simulink model "AI_Compare_2level"  (R2024b)
settings: Solver=ode1  StartTime=0.0  StopTime=4.5  FixedStep=Ts  RelTol=1e-3
PreLoadFcn:
  | Net_improve_init;L=Lac_MV;Tctrl=Ts;
PostLoadFcn:
  | Net_improve_init;L=Lac_MV;Tctrl=Ts;
InitFcn:
  | Net_improve_init;L=Lac_MV;Tctrl=Ts;
undefined symbols (not defined in the file or in its folder): C1, dend, DiscIntNeverNeededParam, f_cari, fs, Lac_MV, numd, Pref, R1, Rac_MV, Ts, Vac_peak_MV, Vdc
libraries: spsControlledVoltageSourceLib x28, powerlib_extras x25, spsGroundLib x14, spsControlledCurrentSourceLib x12, spsCurrentMeasurementLib x11, spsSeriesRLCBranchLib x7, spsThreePhaseVIMeasurementLib x6, spsIdealSwitchLib x5, spsPower3phInstantaneousLib x5, simulink x5, spsVoltageMeasurementLib x3, spsUniversalBridgeLib x1
(part 1 of 4)
Description:
  | The Model initialization function Callback automatically
  | 
  | sets the sample time  to 2e-6 sec.  and loads the initial
  | 
  | states vector xInitial. The initial state vector is saved in the
  | 
  | power_acdrive_init.mat file.
  | 
  | 
  | 
  | Check  the Initial state checkbox in the Simulation
  | 
  | parameters/Workspace I/O to start in steady state with a
  | 
  | speed of 120 rad/s and a torque of 0 N.m/s,
  | 
  | 
  | Copyright 2008-2015 The MathWorks, Inc.
settings Model: Creator=WeiLi  LastModifiedBy=KeXing
settings SolverCC: AlgebraicLoopSolver=TrustRegion
settings DataIOCC: SaveFinalState=on  SaveFormat=Array  SignalLoggingSaveFormat=ModelDataLogs  SaveOutput=off  SaveTime=off  SignalLoggingName=sigsOut
settings OptimizationCC: ExpressionDepthLimit=2147483647  InitFltsAndDblsToZero=on  LifeSpan=inf
settings DebuggingCC: ReadBeforeWriteMsg=DisableAll  WriteAfterWriteMsg=DisableAll  WriteAfterReadMsg=DisableAll  SaveWithParameterizedLinksMsg=none  UnderspecifiedInitializationDetection=Classic  MergeDetectMultiDrivingBlocksExec=none  CheckExecutionContextPreStartOutputMsg=on  MultiTaskDSMMsg=none  MultiTaskCondExecSysMsg=none  FcnCallInpInsideContextMsg=warning  UnconnectedInputMsg=warning  UnconnectedLineMsg=warning  StateNameClashWarn=warning  SFUnexpectedBacktrackingDiag=warning  SFNoUnconditionalDefaultTransitionDiag=warning  SFExecutionAtInitializationDiag=none  ArithmeticOperatorsInVariantConditions=warning
settings HardwareCC: ProdBitPerPointer=32  ProdBitPerSizeT=32  ProdBitPerPtrDiffT=32  ProdLargestAtomicFloat=None  ProdIntDivRoundTo=Undefined  ProdEndianess=Unspecified  ProdWordSize=32  ProdHWDeviceType=32-bit Generic  TargetUnknown=on
settings ModelReferenceCC: UpdateModelReferenceTargets=IfOutOfDate  EnableRefExpFcnMdlSchedulingChecks=on  PropagateSignalLabelsOutOfModel=off
settings SFSimCC: SFSimEcho=off  SimUseLocalCustomCode=off  CustomCodeUndefinedFunction=UseInterfaceOnly
settings RTWCC: RTWUseLocalCustomCode=off  GPUComputeCapability=3.5
settings CodeAppCC: StateflowObjectComments=on
settings GRTTargetCC: TargetFcnLib=ansi_tfl_tmw.mat  TargetLangStandard=C89/C90 (ANSI)  CombineOutputUpdateFcns=off  GRTInterface=on
settings ConfigComp: CovMetricSettings=dw  CovSaveCumulativeToWorkspaceVar=on  CovSaveSingleToWorkspaceVar=on  CovExternalEMLEnable=off
settings SimscapeCC: SimscapeNormalizeSystem=off

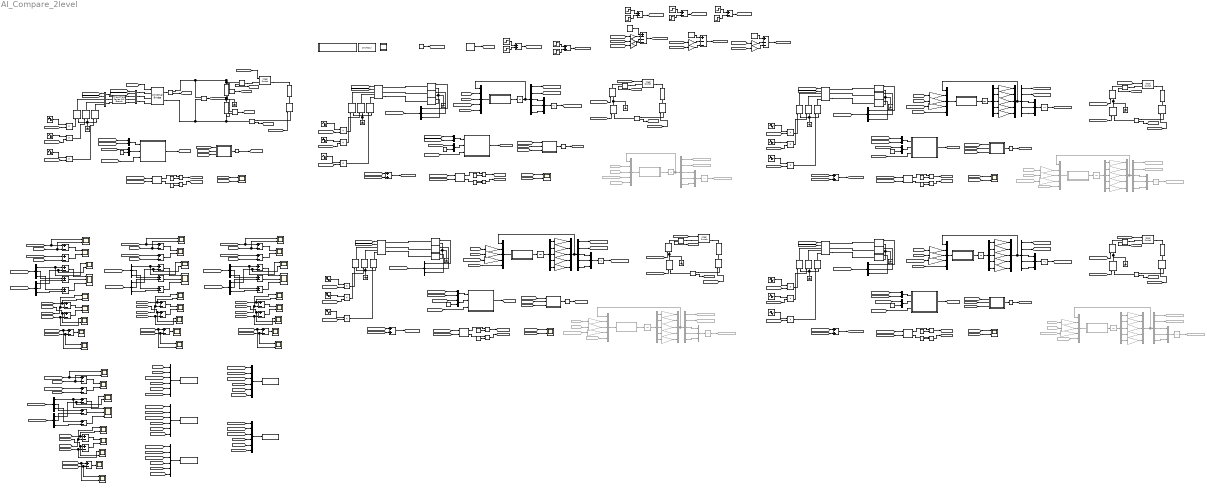
== system AI_Compare_2level ==
  note: Measurment
  note: Open-loop
  note: Close-loop
  note: pHNODE
  note: NODE
  note: Open-loop
  note: Close-loop
  note: pH-NODE vs DUB
  note: NODE vs DUB
  note: Open-loop
  note: LSTM
  note: Close-loop
  note: Close-loop
  note: PINODE
  note: Open-loop
  note: PINODE vs DUB
  note: LSTM vs DUB
  3fault_enable : Sum  Inputs=+-
  Bus_{1..6} (6 alike) : spsThreePhaseVIMeasurementLib/Three-Phase V-I Measurement  VoltageMeasurement=phase-to-ground  SetLabelV=off  LabelV=Vabc  Vpu=off  VpuLL=off  CurrentMeasurement=yes  SetLabelI=off  LabelI=Iabc  Ipu=off  Pbase=P_AC  Vbase=V_AC_prim  OutputType=Complex  PhasorSimulation=off  PSBequivalent=0
  Constant : Constant
  Constant1 : Constant
  Constant2 : Constant
  Controlled Current Source{1..12} (12 alike) : spsControlledCurrentSourceLib/Controlled Current Source  Initialize=on  Source_Type=AC  Amplitude=0  Phase=0  Frequency=0  Measurements=None
  Controlled Voltage Source{1..6,10,20..22,26..28} (13 alike) : spsControlledVoltageSourceLib/Controlled Voltage Source  Initialize=on  Source_Type=DC  Amplitude=3000  Phase=0  Frequency=0  Measurements=None
  Controlled Voltage Source{7..9,11..19,23..25} (15 alike) : spsControlledVoltageSourceLib/Controlled Voltage Source  Initialize=off  Source_Type=AC  Amplitude=0  Phase=0  Frequency=fs  Measurements=None
  Current Measurement{1..11} (11 alike) : spsCurrentMeasurementLib/Current Measurement  PhasorSimulation=off  OutputType=Complex  PSBequivalent=0
  Demux{,7,12,16,23..25} (7 alike) : Demux  Commented=on  Outputs=5
  Demux{1..3,5..6,8,13,17,19..22} (12 alike) : Demux  Outputs=3
  Demux{4,9..11,14..15,18} (7 alike) : Demux  Outputs=5
  Divide{1..10} (10 alike) : Product  Inputs=*/
  From115 : From  Commented=on  GotoTag=Idc_Ld5
  From117 : From  Commented=on  GotoTag=Idc_Ld6
  From119 : From  Commented=on  GotoTag=Vabc_Bus_MV3
  From{93,123,138,165} (4 alike) : From  Commented=on  GotoTag=pulses1
  From129 : From  Commented=on  GotoTag=Idc_Ld7
  From131 : From  Commented=on  GotoTag=Idc_Ld8
  From133 : From  Commented=on  GotoTag=Vabc_Bus_MV4
  From156 : From  Commented=on  GotoTag=Idc_Ld9
  From158 : From  Commented=on  GotoTag=Idc_Ld10
  From160 : From  Commented=on  GotoTag=Vabc_Bus_MV5
  From45 : From  Commented=on  GotoTag=Idc_Ld3
  From58 : From  Commented=on  GotoTag=Idc_Ld4
  From60 : From  Commented=on  GotoTag=Vabc_Bus_MV2
  Gain{,1..3} (4 alike) : Gain  Gain=0.9
  Gain10 : Gain  Gain=1811.85
  Gain11 : Gain  Gain=1795.81
  Gain12 : Gain  Gain=186.98
  Gain13 : Gain  Gain=193.63
  Gain14 : Gain  Gain=187.97
  Gain15 : Gain  Gain=1811.85
  Gain16 : Gain  Gain=1795.81
  Gain17 : Gain  Gain=186.98
  Gain18 : Gain  Gain=193.63
  Gain19 : Gain  Gain=187.97
  Gain{7,9,20,22,28,30} (6 alike) : Gain  Gain=1/116.32
  Gain21 : Gain  Gain=1/1405.94
  Gain23 : Gain  Commented=on  Gain=1811.85
  Gain24 : Gain  Commented=on  Gain=1795.81
  Gain25 : Gain  Commented=on  Gain=186.98
  Gain26 : Gain  Commented=on  Gain=193.63
  Gain27 : Gain  Commented=on  Gain=187.97
  Gain29 : Gain  Gain=1/1405.94
  Gain{31,33,39,41,47,49} (6 alike) : Gain  Commented=on  Gain=1/116.32
  Gain32 : Gain  Commented=on  Gain=1/1405.94
  Gain34 : Gain  Commented=on  Gain=1811.85
  Gain35 : Gain  Commented=on  Gain=1795.81
  Gain36 : Gain  Commented=on  Gain=186.98
  Gain37 : Gain  Commented=on  Gain=193.63
  Gain38 : Gain  Commented=on  Gain=187.97
  Gain4 : Gain  Gain=0.2
  Gain40 : Gain  Commented=on  Gain=1/1405.94
  Gain42 : Gain  Commented=on  Gain=1811.85
  Gain43 : Gain  Commented=on  Gain=1795.81
  Gain44 : Gain  Commented=on  Gain=186.98
  Gain45 : Gain  Commented=on  Gain=193.63
  Gain46 : Gain  Commented=on  Gain=187.97
  Gain48 : Gain  Commented=on  Gain=1/1405.94
  Gain5 : Gain  Gain=0.2
  Gain55 : Gain  Gain=1811.85
  Gain56 : Gain  Gain=1795.81
  Gain57 : Gain  Gain=186.98
  Gain58 : Gain  Gain=193.63
  Gain59 : Gain  Gain=187.97
  Gain6 : Gain  Gain=0.2
  Gain8 : Gain  Gain=1/1405.94
  Goto11 : Goto  Commented=on  GotoTag=Iabc_pred2
  Goto12 : Goto  Commented=on  GotoTag=vcp_pred3
  Goto13 : Goto  Commented=on  GotoTag=vcn_pred3
  Goto2 : Goto  Commented=on  GotoTag=Iabc_pred3
  Goto22 : Goto  Commented=on  GotoTag=vcp_pred2
  Goto23 : Goto  Commented=on  GotoTag=vcn_pred2
  Goto55 : Goto  Commented=on  GotoTag=Iabc_pred4
  Goto56 : Goto  Commented=on  GotoTag=vcp_pred4
  Goto61 : Goto  Commented=on  GotoTag=vcn_pred4
  Goto71 : Goto  Commented=on  GotoTag=Iabc_pred5
  Goto72 : Goto  Commented=on  GotoTag=vcp_pred5
  Goto76 : Goto  Commented=on  GotoTag=vcn_pred5
  Ground{1..14} (14 alike) : spsGroundLib/Ground  LConnTagsString=a
  Help : Subsystem  mask(OpDoc){docfile=../Help/help.html}
      mask init:
      | %patch([1,1,0,0,.8,1],[.8,0,0,1,1,.8],[.8 .8 .8]);
      | %patch([.15 .78 .78 .15 .15],[.8 .8 .83 .83 .8],[.9 .9 .9]);
      | %patch([.15 .78 .78 .15 .15],[.7 .7 .73 .73 .8],[.9 .9 .9]);
      | %patch([.15 .78 .78 .15 .15],[.6 .6 .63 .63 .6],[.9 .9 .9]);
      | %patch([.15 .78 .78 .15 .15],[.5 .5 .53 .53 .5],[.9 .9 .9]);
      | %patch([.15 .78 .78 .15 .15],[.4 .4 .43 .43 .4],[.9 .9 .9]);
      settings: OpenFcn=OpHelp_cb(gcb);
      mask Display: image(imread('opdoc.bmp'))
  IGBT Inverter2 : spsUniversalBridgeLib/Universal Bridge  Arms=3  SnubberResistance=IGBT_Rs  SnubberCapacitance=1e-6  Device=IGBT / Diodes  Ron=IGBT_Ron  Lon=0  ForwardVoltages=[0 0]  ForwardVoltage=.8  GTOparameters=[ 1e-6 , 1e-6 ]  IGBTparameters=[0 0]  Measurements=Device voltages  Measurements_2=None  converterType=Rectifier
      settings: AttributesFormatString=\n
  Ideal Switch{1..5} (5 alike) : spsIdealSwitchLib/Ideal Switch  Ron=0.001  Lon=0  IC=0  Rs=1e9  Cs=inf  Measurements=on
  Integrator : Integrator  Commented=on
  Integrator1 : Integrator
  Integrator2 : Integrator  Commented=on
  Integrator3 : Integrator  InitialCondition=1
  Integrator4 : Integrator  Commented=on
  Integrator7 : Integrator
  MATLAB Function : MATLAB Function  Commented=on  TreatAsAtomicUnit=on
  MATLAB Function1 : MATLAB Function  TreatAsAtomicUnit=on
  MATLAB Function2 : MATLAB Function  Commented=on  TreatAsAtomicUnit=on
  MATLAB Function3 : MATLAB Function  TreatAsAtomicUnit=on
  MATLAB Function4 : MATLAB Function  Commented=on  TreatAsAtomicUnit=on
  MATLAB Function5 : MATLAB Function  TreatAsAtomicUnit=on
  MATLAB Function6 : MATLAB Function  Commented=on  TreatAsAtomicUnit=on
  MATLAB Function7 : MATLAB Function  TreatAsAtomicUnit=on
  Memory{1..5} (5 alike) : Memory
  Minus{1..3,5} (4 alike) : Sum
  Model Initialization : Subsystem  mask(Model Functions){InitFcnX=Net_improve_init;L=Lac_MV;Tctrl=Ts;, prel=on, posl=on, inif=on, strf=off}
      mask prompts: InitFcnX "Initialisation"; prel "Preload Function"; posl "PostLoad Function"; inif "InitFcn"; strf "StartFcn"
      mask init:
      | currentBlock = gcb;
      | root = bdroot(currentBlock);
      | 
      | if ~strcmp(get_param(root,'BlockDiagramType'),'library')
      |     if prel==1
      |         set_param(root, 'PreLoadFcn', InitFcnX);
      |     else
      |         set_param(root, 'PreLoadFcn', '');
      |     end
      |     if inif==1
      |         set_param(root, 'InitFcn', InitFcnX);
      |     else
      |         set_param(root, 'InitFcn', '');
      |     end
      |     if strf==1
      |         set_param(root, 'StartFcn', InitFcnX);
      |     else
      |         set_param(root, 'StartFcn', '');
      |     end
      |     if posl==1
      |         set_param(root, 'PostLoadFcn', InitFcnX);
      |     else
      |         set_param(root, 'PostLoadFcn', '');
      |     end
      | end
      | 
      | pos = get_param(currentBlock, 'Position');
      | width = pos(3) - pos(1); height = pos(4) - pos(2);
      | txt = [ upper(root) '\n' '- InitFcn. . . . . '  get_param(root, 'InitFcn') ];
      settings: CopyFcn=set_param(gcb,'LinkStatus','none')
      mask Display: text(5, height*0.5, txt, 'horizontalAlignment', 'left', 'verticalAlignment', 'middle') ;
  Mux{,9,24,31} (4 alike) : Mux  Commented=on  Inputs=3
  Mux{1,10,18,25,34..36} (7 alike) : Mux  Commented=on  Inputs=5
  Mux{4..5,8,11,13..14,19..20,26..27} (10 alike) : Mux  Inputs=2
  Mux{2..3,12,32..33} (5 alike) : Mux  Inputs=6
  Mux{6,15,21,28} (4 alike) : Mux  Inputs=3
  Mux{7,16..17,22..23,29..30} (7 alike) : Mux  Inputs=5
  PWM_SPS1 : Subsystem
  PWM_SPS2 : Subsystem
  PWM_SPS3 : Subsystem
  PWM_SPS4 : Subsystem
  PWM_SPS5 : Subsystem
  P_AE{,1..3} (4 alike) : Sum  Inputs=+-
  Power (3ph, Instantaneous){1..5} (5 alike) : spsPower3phInstantaneousLib/Power (3ph, Instantaneous)
  Product{1..15} (15 alike) : Product
  Pstep : Sum
  Pstep1 : Sum
  Q_AE{,1..3} (4 alike) : Sum  Inputs=+-
  Qref_pu{1..5,7,10..11,13..14} (10 alike) : Constant  Value=Pref
  Qref_pu{6,8..9,12,15} (5 alike) : Constant  Value=0
  Rec_VQcontrol1 : Subsystem  mask(converter controller){cm=off, base=[Pref, Vac_peak_MV*sqrt(3/2), Vdc/2, fs], LRx=[Lac_MV, Rac_MV], LRx_inpu=off, Kd=[0.3  2]*10/6  %was [1 0.1]   ; [0.1  1]*1, Kp=[0.3 1]*1     %was [1 0.1]   ; [0.1  1]*1, Kvdc=[2 10]*1;   %was [0.5 1]*20 for Cdc=320uF, Vabc_lim=[-1 1], limitVdq=1.1, nadv=6, xtrIctrl1=[0.4 10 10 -10], Ts=Tctrl}
      mask prompts: cm "control mode (check VQ/uncheck PQ), only one terminal in VQ mode"; base "base value for power(VA), ac voltage(V), dc voltage to ground(V), and frequenvy(Hz) [Sb, Vb, Vdcb,freq]"; LRx "commutation inductance and resistance [Lx, Rx]"; LRx_inpu "[Lx, Rx] in pu if checked/ SI unchecked"; Kd "Kp Ki for d-axis PI control [kp ki]"; Kp "Kp Ki for q-axis PI control [kp ki]"; Kvdc "Kp Ki for Vdc PI control [kp ki]"; Vabc_lim "output Vabc limit [min max]"; limitVdq "limit for Vd,Vq (pu, default = 1.1)"; nadv "nb of time step to compesate for delay (default=1)"; xtrIctrl1 "[kp, kp, limitmax, limitmin] for current control (default=[0.4, 10, 10, -10])"
      mask help:
      | input 1, 6 dimentions, Vabc, Iabc, (SI)
      | input 2, 2 dimentions, Pref, Qref (PU)
      | input 3, 6 dimentions, Vcap at up arm a, lower arm a, up arm b, lower arm b, up arm c and lower arm c.
      | input 4, 1 dimention, pulse on
      | input 5, 1 dimention
      |
      | power or current directions: to go into grid is positive
      mask init:
      | if cm==0;
      |     x=['PQ\nmode'];
      | else
      |     x=['VQ\nmode'];
      | end
      | 
      | Sb=base(1);            %VA 3phase power base;
      | Vb=base(2);       %V, line-line rms voltage base
      | Ib=Sb/(sqrt(3)*Vb); %A, rms current base
      | Zb=Vb^2/Sb ;        %ohm, impedence base
      | Vdc=base(3);      %V Vdc+ to ground or ground to Vdc- 
      | frq=base(4);
      | 
      | if LRx_inpu
      |     Rxpu=LRx(2);
      |     Lxpu=LRx(1);
      | else
      |     Rxpu=LRx(2)/Zb;
      |     Lxpu=LRx(1)*2*pi*frq/Zb;
      | end;
      | 
      | ks=Vdc*sqrt(3/2)/Vb;     % ma=1/ks for 1pu dc ->1pu ac;
      | 
      | Kp=Kd;
      mask DialogControl ParameterTabVar0 Prompt: parameters
      mask DialogControl ParameterTabVar01 Prompt: advanced
      mask Display: disp (x);
  Rec_VQcontrol2 : Subsystem  mask(converter controller){cm=off, base=[Pref, Vac_peak_MV*sqrt(3/2), Vdc/2, fs], LRx=[Lac_MV, Rac_MV], LRx_inpu=off, Kd=[0.3  2]*10/6  %was [1 0.1]   ; [0.1  1]*1, Kp=[0.3 1]*1     %was [1 0.1]   ; [0.1  1]*1, Kvdc=[2 10]*1;   %was [0.5 1]*20 for Cdc=320uF, Vabc_lim=[-1 1], limitVdq=1.1, nadv=6, xtrIctrl1=[0.4 10 10 -10], Ts=Tctrl}
      mask prompts: cm "control mode (check VQ/uncheck PQ), only one terminal in VQ mode"; base "base value for power(VA), ac voltage(V), dc voltage to ground(V), and frequenvy(Hz) [Sb, Vb, Vdcb,freq]"; LRx "commutation inductance and resistance [Lx, Rx]"; LRx_inpu "[Lx, Rx] in pu if checked/ SI unchecked"; Kd "Kp Ki for d-axis PI control [kp ki]"; Kp "Kp Ki for q-axis PI control [kp ki]"; Kvdc "Kp Ki for Vdc PI control [kp ki]"; Vabc_lim "output Vabc limit [min max]"; limitVdq "limit for Vd,Vq (pu, default = 1.1)"; nadv "nb of time step to compesate for delay (default=1)"; xtrIctrl1 "[kp, kp, limitmax, limitmin] for current control (default=[0.4, 10, 10, -10])"
      mask help:
      | input 1, 6 dimentions, Vabc, Iabc, (SI)
      | input 2, 2 dimentions, Pref, Qref (PU)
      | input 3, 6 dimentions, Vcap at up arm a, lower arm a, up arm b, lower arm b, up arm c and lower arm c.
      | input 4, 1 dimention, pulse on
      | input 5, 1 dimention
      |
      | power or current directions: to go into grid is positive
      mask init: same as AI_Compare_2level/Rec_VQcontrol1
      mask DialogControl ParameterTabVar0 Prompt: parameters
      mask DialogControl ParameterTabVar01 Prompt: advanced
      mask Display: disp (x);
  Rec_VQcontrol3 : Subsystem  mask(converter controller){cm=off, base=[Pref, Vac_peak_MV*sqrt(3/2), Vdc/2, fs], LRx=[Lac_MV, Rac_MV], LRx_inpu=off, Kd=[0.3  2]*10/6  %was [1 0.1]   ; [0.1  1]*1, Kp=[0.3 1]*1     %was [1 0.1]   ; [0.1  1]*1, Kvdc=[2 10]*1;   %was [0.5 1]*20 for Cdc=320uF, Vabc_lim=[-1 1], limitVdq=1.1, nadv=6, xtrIctrl1=[0.4 10 10 -10], Ts=Tctrl}
      mask prompts: cm "control mode (check VQ/uncheck PQ), only one terminal in VQ mode"; base "base value for power(VA), ac voltage(V), dc voltage to ground(V), and frequenvy(Hz) [Sb, Vb, Vdcb,freq]"; LRx "commutation inductance and resistance [Lx, Rx]"; LRx_inpu "[Lx, Rx] in pu if checked/ SI unchecked"; Kd "Kp Ki for d-axis PI control [kp ki]"; Kp "Kp Ki for q-axis PI control [kp ki]"; Kvdc "Kp Ki for Vdc PI control [kp ki]"; Vabc_lim "output Vabc limit [min max]"; limitVdq "limit for Vd,Vq (pu, default = 1.1)"; nadv "nb of time step to compesate for delay (default=1)"; xtrIctrl1 "[kp, kp, limitmax, limitmin] for current control (default=[0.4, 10, 10, -10])"
      mask help:
      | input 1, 6 dimentions, Vabc, Iabc, (SI)
      | input 2, 2 dimentions, Pref, Qref (PU)
      | input 3, 6 dimentions, Vcap at up arm a, lower arm a, up arm b, lower arm b, up arm c and lower arm c.
      | input 4, 1 dimention, pulse on
      | input 5, 1 dimention
      |
      | power or current directions: to go into grid is positive
      mask init: same as AI_Compare_2level/Rec_VQcontrol1
      mask DialogControl ParameterTabVar0 Prompt: parameters
      mask DialogControl ParameterTabVar01 Prompt: advanced
      mask Display: disp (x);
  Rec_VQcontrol4 : Subsystem  mask(converter controller){cm=off, base=[Pref, Vac_peak_MV*sqrt(3/2), Vdc/2, fs], LRx=[Lac_MV, Rac_MV], LRx_inpu=off, Kd=[0.3  2]*10/6  %was [1 0.1]   ; [0.1  1]*1, Kp=[0.3 1]*1     %was [1 0.1]   ; [0.1  1]*1, Kvdc=[2 10]*1;   %was [0.5 1]*20 for Cdc=320uF, Vabc_lim=[-1 1], limitVdq=1.1, nadv=6, xtrIctrl1=[0.4 10 10 -10], Ts=Tctrl}
      mask prompts: cm "control mode (check VQ/uncheck PQ), only one terminal in VQ mode"; base "base value for power(VA), ac voltage(V), dc voltage to ground(V), and frequenvy(Hz) [Sb, Vb, Vdcb,freq]"; LRx "commutation inductance and resistance [Lx, Rx]"; LRx_inpu "[Lx, Rx] in pu if checked/ SI unchecked"; Kd "Kp Ki for d-axis PI control [kp ki]"; Kp "Kp Ki for q-axis PI control [kp ki]"; Kvdc "Kp Ki for Vdc PI control [kp ki]"; Vabc_lim "output Vabc limit [min max]"; limitVdq "limit for Vd,Vq (pu, default = 1.1)"; nadv "nb of time step to compesate for delay (default=1)"; xtrIctrl1 "[kp, kp, limitmax, limitmin] for current control (default=[0.4, 10, 10, -10])"
      mask help:
      | input 1, 6 dimentions, Vabc, Iabc, (SI)
      | input 2, 2 dimentions, Pref, Qref (PU)
      | input 3, 6 dimentions, Vcap at up arm a, lower arm a, up arm b, lower arm b, up arm c and lower arm c.
      | input 4, 1 dimention, pulse on
      | input 5, 1 dimention
      |
      | power or current directions: to go into grid is positive
      mask init: same as AI_Compare_2level/Rec_VQcontrol1
      mask DialogControl ParameterTabVar0 Prompt: parameters
      mask DialogControl ParameterTabVar01 Prompt: advanced
      mask Display: disp (x);
  Rec_VQcontrol5 : Subsystem  mask(converter controller){cm=off, base=[Pref, Vac_peak_MV*sqrt(3/2), Vdc/2, fs], LRx=[Lac_MV, Rac_MV], LRx_inpu=off, Kd=[0.3  2]*10/6  %was [1 0.1]   ; [0.1  1]*1, Kp=[0.3 1]*1     %was [1 0.1]   ; [0.1  1]*1, Kvdc=[2 10]*1;   %was [0.5 1]*20 for Cdc=320uF, Vabc_lim=[-1 1], limitVdq=1.1, nadv=6, xtrIctrl1=[0.4 10 10 -10], Ts=Tctrl}
      mask prompts: cm "control mode (check VQ/uncheck PQ), only one terminal in VQ mode"; base "base value for power(VA), ac voltage(V), dc voltage to ground(V), and frequenvy(Hz) [Sb, Vb, Vdcb,freq]"; LRx "commutation inductance and resistance [Lx, Rx]"; LRx_inpu "[Lx, Rx] in pu if checked/ SI unchecked"; Kd "Kp Ki for d-axis PI control [kp ki]"; Kp "Kp Ki for q-axis PI control [kp ki]"; Kvdc "Kp Ki for Vdc PI control [kp ki]"; Vabc_lim "output Vabc limit [min max]"; limitVdq "limit for Vd,Vq (pu, default = 1.1)"; nadv "nb of time step to compesate for delay (default=1)"; xtrIctrl1 "[kp, kp, limitmax, limitmin] for current control (default=[0.4, 10, 10, -10])"
      mask help:
      | input 1, 6 dimentions, Vabc, Iabc, (SI)
      | input 2, 2 dimentions, Pref, Qref (PU)
      | input 3, 6 dimentions, Vcap at up arm a, lower arm a, up arm b, lower arm b, up arm c and lower arm c.
      | input 4, 1 dimention, pulse on
      | input 5, 1 dimention
      |
      | power or current directions: to go into grid is positive
      mask init: same as AI_Compare_2level/Rec_VQcontrol1
      mask DialogControl ParameterTabVar0 Prompt: parameters
      mask DialogControl ParameterTabVar01 Prompt: advanced
      mask Display: disp (x);
  Scope{1..2,4..9,11..13,15..19,21..23,25..27,29..32,34..36,38..41} (33 alike) : Scope  NumInputPorts=2
  Scope{10,14,24,33} (4 alike) : Scope
  Scope{3,20,28,37} (4 alike) : Scope  NumInputPorts=3
  Series RLC Branch{1..2,4,6..7} (5 alike) : spsSeriesRLCBranchLib/Series RLC Branch  LConnTagsString=__new0  RConnTagsString=__new0  BranchType=R  Resistance=3e3^2/(Pref)/10*2  Inductance=1e-3  SetiL0=off  InitialCurrent=0  Capacitance=C1  Setx0=off  InitialVoltage=0  Measurements=None
  Series RLC Branch3 : spsSeriesRLCBranchLib/Series RLC Branch  LConnTagsString=__new0  RConnTagsString=__new0  BranchType=C  Resistance=R1  Inductance=1e-3  SetiL0=off  InitialCurrent=0  Capacitance=C1  Setx0=off  InitialVoltage=0  Measurements=None
  Series RLC Branch5 : spsSeriesRLCBranchLib/Series RLC Branch  LConnTagsString=__new0  RConnTagsString=__new0  BranchType=C  Resistance=R1  Inductance=1e-3  SetiL0=off  InitialCurrent=0  Capacitance=C1  Setx0=off  InitialVoltage=0  Measurements=None
  Sine Wave{1,3,6,10,13} (5 alike) : Sin  Amplitude=3e3/2*sqrt(2/3)  Frequency=2*pi*fs  SampleTime=0
  Sine Wave{2,4,7,11,14} (5 alike) : Sin  Amplitude=3e3/2*sqrt(2/3)  Frequency=2*pi*fs  Phase=-2*pi/3  SampleTime=0
  Sine Wave{5,8..9,12,15} (5 alike) : Sin  Amplitude=3e3/2*sqrt(2/3)  Frequency=2*pi*fs  Phase=+2*pi/3  SampleTime=0
  Step1 : Step  Time=2.75  Before=-0.8  After=-0.6  SampleTime=0
  Step10 : Step  Time=3.85  SampleTime=0
  Step2 : Step  Time=3.25  Before=3000  After=2400  SampleTime=0
  Step3 : Step  Time=3.0  Before=0.0  After=-0.2  SampleTime=0
  Step4 : Step  Time=1.75  Before=1.9  SampleTime=0
  Step5 : Step  Time=3.5  After=600  SampleTime=0
  Step6 : Step  Time=1.65  SampleTime=0
  Step7 : Step  Time=2.5  SampleTime=0
  Step8 : Step  Time=2.65  SampleTime=0
  Step9 : Step  Time=3.70  SampleTime=0
  Three-Phase RL1 : spsThreePhaseSeriesRLCBranchLib/Three-Phase Series RLC Branch  LConnTagsString=A|B|C  RConnTagsString=A|B|C  BranchType=RL  Resistance=Rac_MV  Inductance=Lac_MV  Capacitance=1e-6  Measurements=None
  To Workspace : ToWorkspace  VariableName=z_pq_phnode  SampleTime=-1
      settings: Save2DSignal=2-D array (concatenate along first dimension)
  To Workspace1 : ToWorkspace  VariableName=z_pq_dub  SampleTime=-1
      settings: Save2DSignal=2-D array (concatenate along first dimension)
  To Workspace2 : ToWorkspace  VariableName=z_pq_node  SampleTime=-1
      settings: Save2DSignal=2-D array (concatenate along first dimension)
  To Workspace3 : ToWorkspace  VariableName=z_pq_lstm  SampleTime=-1
      settings: Save2DSignal=2-D array (concatenate along first dimension)
  To Workspace4 : ToWorkspace  VariableName=z_pq_pinode  SampleTime=-1
      settings: Save2DSignal=2-D array (concatenate along first dimension)
  Unary Minus{1,3,5,7} (4 alike) : UnaryMinus  Commented=on
  Unary Minus{2,4,6,8} (4 alike) : UnaryMinus
  Unit Delay : UnitDelay  SampleTime=-1  HasFrameUpgradeWarning=on
  Unit Delay1 : UnitDelay  Commented=on  SampleTime=-1  HasFrameUpgradeWarning=on
  Voltage Measurement1 : spsVoltageMeasurementLib/Voltage Measurement  PhasorSimulation=off  OutputType=Complex  PSBequivalent=0
  Voltage Measurement2 : spsVoltageMeasurementLib/Voltage Measurement  PhasorSimulation=off  OutputType=Complex  PSBequivalent=0
  Voltage Measurement3 : spsVoltageMeasurementLib/Voltage Measurement  PhasorSimulation=off  OutputType=Complex  PSBequivalent=0
  afault_enable1 : Sum  Inputs=+-
  afault_enable2 : Sum  Inputs=+-
  carrier gen1 : libMMCcpuv2/carrier gen  fc=f_cari*2  range=[ 1 -1]  Ms=3  Ns=1
  ia_AE{,1..3} (4 alike) : Sum  Inputs=+-
  ib_AE{,1..3} (4 alike) : Sum  Inputs=+-
  ic_AE{,1..3} (4 alike) : Sum  Inputs=+-
  ka : Sum  Inputs=+---
  kb : Sum  Inputs=+--
  kb1 : Sum  Inputs=+--
  powergui : spspowerguiLib/powergui  Priority=2  SimulationMode=Discrete  SampleTime=Ts  frequency=60  Iterations=50  frequencyindice=0  Pbase=100e6  ErrMax=1e-4  UnitsV=kV  UnitsW=MW  buscounter=0  FunctionMessages=off  echomessages=off  EnableUseOfTLC=off  CurrentSourceSwitches=off  DisableSnubberDevices=off  DisableRonSwitches=off  DisableVfSwitches=off  DisplayEquations=off  AutomaticDiscreteSolvers=off  SolverType=Backward Euler  Interpol=off  ExternalGateDelay=off  methode=off  Ts=0  x0status=blocks  SPID=off  SwTol=0  HookPort=off  NonlinearTolerance=1e-4  nMaxIteration=100  ContinueOnMaxIteration=off  RestoreLinks=warning  ResistiveCurrentMeasurement=off  Frange=[0:2:500]  Ylog=off  Xlog=on  ShowGrid=off  save=off  variable=ZData  structure=VI  ZoomFFT=off  StartTime=9  cycles=10  DisplayStyle=2  fundamental=300/pi  FreqAxis=off  MaxFrequency=1000  frequencyindicesteady=1  RmsSteady=1  display=off
  pulse_enable : Constant
  vcn_AE{,1..3} (4 alike) : Sum  Inputs=+-
  vcp_AE{,1..7} (8 alike) : Sum  Inputs=+-
  wires:
  carrier gen1/1 -> [pwmcarrier]
  [pulse_enable] -> PWM_SPS3/1(enable)
  Mux4/1 -> Rec_VQcontrol2/1(meas)
  Mux5/1 -> Rec_VQcontrol2/2(PQref)
  Qref_pu6/1 -> Mux5/2
  [power_step] -> Mux5/1
  pulse_enable/1 -> [pulse_enable]
  PWM_SPS3/1(Pulse) -> Memory2/1
  Rec_VQcontrol2/1(V_cell_ref) -> [Vref_PQctrl2]
  Memory2/1 -> [pulses2]
  [Iabc_Bus_MV1] -> Demux1/1
  vcp_AE/1 -> Scope2/1
  vcn_AE/1 -> Scope2/2
  ib_AE/1 -> Scope3/2
  ic_AE/1 -> Scope3/3
  Step1/1 -> Pstep/1
  Bus_2/1 -> [Vabc_Bus_MV2]
  Bus_2/2 -> [Iabc_Bus_MV2]
  [pulse_enable] -> Ideal Switch1/1
  Current Measurement2/1 -> [Idc_Ld3]
  Current Measurement4/1 -> [Idc_Ld4]
  [vcp_pred2] -> Controlled Voltage Source1/1
  [vcn_pred2] -> Controlled Voltage Source5/1
  Minus5/1 -> [Vdc_pred2]
  [vcp_pred2] -> Minus5/1
  [vcn_pred2] -> Minus5/2
  Demux1/2 -> ib_AE/2
  Demux1/3 -> ic_AE/2
  Demux3/1 -> Scope13/1, ia_AE/1
  Demux3/2 -> ib_AE/1
  Demux3/3 -> ic_AE/1
  [Iabc_pred2] -> Demux3/1
  [Vcp1] -> Scope4/2, vcp_AE/2
  [Vcn1] -> vcn_AE/2
  [vcp_pred2] -> Scope4/1, vcp_AE/1
  [vcn_pred2] -> vcn_AE/1
  "Power (3ph, Instantaneous)1"/1 -> Divide2/1
  Qref_pu4/1 -> Divide3/2
  Qref_pu3/1 -> Divide2/2
  "Power (3ph, Instantaneous)1"/2 -> Divide3/1
  Divide2/1 -> [P2]
  Divide3/1 -> [Q2]
  [P2] -> Scope8/1
  [Q2] -> Scope8/2
  [Vabc_Bus_MV2] -> "Power (3ph, Instantaneous)1"/1
  [Iabc_Bus_MV2] -> "Power (3ph, Instantaneous)1"/2
  Integrator/1 -> Mux1/1, Demux/1
  [Iabc_pred2] -> Demux2/1
  Demux2/1 -> Controlled Current Source2/1
  Demux2/2 -> Controlled Current Source1/1
  Demux2/3 -> Controlled Current Source3/1
  [P1] -> Scope11/2, P_AE/1
  [P2] -> P_AE/2, Scope11/1
  [Q1] -> Scope17/2, Q_AE/1
  [Q2] -> Scope17/1, Q_AE/2
  P_AE/1 -> Scope1/1
  Q_AE/1 -> Scope1/2
  ia_AE/1 -> Scope3/1
  Demux1/1 -> Scope13/2, ia_AE/2
  [vcp_pred2] -> Mux2/1
  [vcn_pred2] -> Mux2/2
  [Iabc_pred2] -> Mux2/3
  [P2] -> Mux2/4
  [Q2] -> Mux2/5
  Mux2/1 -> To Workspace/1
  [Vcp1] -> Mux3/1
  [Vcn1] -> Mux3/2
  [Iabc_Bus_MV1] -> Mux3/3
  [P1] -> Mux3/4
  [Q1] -> Mux3/5
  Mux3/1 -> To Workspace1/1
  [Idc_Ld3] -> Mux7/2
  Integrator1/1 -> Mux7/1, Demux4/1
  [Idc_Ld4] -> Mux7/3
  Demux4/2 -> [vcn_pred2]  "vcn"
  Unary Minus2/1 -> [Iabc_pred2]
  MATLAB Function1/1(dz) -> Integrator1/1
  [Vabc_Bus_MV2] -> Mux7/4
  Mux7/1 -> MATLAB Function1/1(u)
  Demux4/5 -> Mux6/3  "ic"
  Mux6/1 -> Unary Minus2/1
  Demux4/1 -> [vcp_pred2]  "vcp"
  Demux4/4 -> Mux6/2  "ib"
  Demux4/3 -> Mux6/1  "ia"
  From45/1 -> Mux1/2
  From58/1 -> Mux1/3
  From60/1 -> Mux1/4
  From93/1 -> Mux1/5
  MATLAB Function/1(dz) -> Integrator/1
  Demux/1 -> Goto22/1  "vcp"
  Demux/2 -> Goto23/1  "vcn"
  Demux/3 -> Mux/1  "ia"
  Demux/4 -> Mux/2  "ib"
  Demux/5 -> Mux/3  "ic"
  Mux/1 -> Unary Minus1/1
  Unary Minus1/1 -> Goto11/1
  Mux1/1 -> MATLAB Function/1(u)
  [dc_step] -> Controlled Voltage Source2/1
  Sine Wave5/1 -> Product5/1
  Sine Wave3/1 -> Product3/1
  [ac_step_c] -> Product5/2
  Sine Wave4/1 -> Product4/1
  [ac_step_b] -> Product4/2
  [ac_step_a] -> Product3/2
  Product3/1 -> Controlled Voltage Source7/1
  Product4/1 -> Controlled Voltage Source8/1
  Product5/1 -> Controlled Voltage Source9/1
  [Iabc_Bus_MV2] -> Mux4/2
  [Vref_PQctrl2] -> PWM_SPS3/2(Vref)
  [pwmcarrier] -> PWM_SPS3/3(pwmcarrier)
  [Vabc_Bus_MV2] -> Mux4/1
  [Vdc_pred2] -> Rec_VQcontrol2/3(Vdc)
  [Vdc_pred2] -> Scope15/2, vcp_AE6/1
  [Vdc_meas1] -> Scope15/1, vcp_AE6/2
  vcp_AE6/1 -> Scope14/1
  [Vdc_pred2] -> Mux2/6
  [Vdc_meas1] -> Mux3/6
  [pulses2] -> Mux7/5
  [Vabc_Bus_MV1] -> "Power (3ph, Instantaneous)2"/1
  Qref_pu7/1 -> Divide5/2
  [Iabc_Bus_MV1] -> "Power (3ph, Instantaneous)2"/2
  Mux8/1 -> Rec_VQcontrol3/2(PQref)
  Divide5/1 -> [Q1]
  Rec_VQcontrol3/1(V_cell_ref) -> [Vref_PQctrl1]
  [power_step] -> Mux8/1
  Voltage Measurement1/1 -> [Vcp1]
  Sine Wave7/1 -> Product7/1
  Qref_pu9/1 -> Mux8/2
  [dc_step] -> Controlled Voltage Source10/1
  Voltage Measurement3/1 -> [Vdc_meas1]
  [Iabc_Bus_MV1] -> Mux11/2
  Sine Wave8/1 -> Product8/1
  Memory3/1 -> [pulses1]
  [P1] -> Scope12/1
  Bus_5/1 -> [Vabc_con_MV1]
  Current Measurement8/1 -> [Idc_Ld2]
  Voltage Measurement2/1 -> [Vcn1]
  Sine Wave6/1 -> Product6/1
  Product6/1 -> Controlled Voltage Source11/1
  [pulses1] -> IGBT Inverter2/1
  Bus_3/2 -> [Iabc_Bus_MV1]
  [Vabc_Bus_MV1] -> Mux11/1
  [ac_step_c] -> Product8/2
  [pulse_enable] -> PWM_SPS2/1(enable)
  [Vdc_meas1] -> Rec_VQcontrol3/3(Vdc)
  Current Measurement6/1 -> [Idc_meas1]
  Mux11/1 -> Rec_VQcontrol3/1(meas)
  [ac_step_b] -> Product7/2
  "Power (3ph, Instantaneous)2"/2 -> Divide5/1
  [pwmcarrier] -> PWM_SPS2/3(pwmcarrier)
  [pulse_enable] -> Ideal Switch3/1
  Current Measurement7/1 -> [Idc_Ld1]
  Product8/1 -> Controlled Voltage Source13/1
  "Power (3ph, Instantaneous)2"/1 -> Divide4/1
  [Q1] -> Scope12/2
  [Vref_PQctrl1] -> PWM_SPS2/2(Vref)
  Divide4/1 -> [P1]
  Qref_pu5/1 -> Divide4/2
  Bus_3/1 -> [Vabc_Bus_MV1]
  Bus_5/2 -> [iabc_con_MV1]
  [ac_step_a] -> Product6/2
  Product7/1 -> Controlled Voltage Source12/1
  PWM_SPS2/1(Pulse) -> Memory3/1
  [P1] -> Scope7/2, P_AE1/1
  P_AE1/1 -> Scope5/1
  vcn_AE1/1 -> Scope19/2
  Demux6/1 -> Scope9/1, ia_AE1/1
  Demux5/1 -> Scope9/2, ia_AE1/2
  Demux5/3 -> ic_AE1/2
  Demux5/2 -> ib_AE1/2
  [Q1] -> Scope18/2, Q_AE1/1
  vcp_AE1/1 -> Scope19/1
  [Iabc_pred3] -> Demux6/1
  [Iabc_Bus_MV1] -> Demux5/1
  ic_AE1/1 -> Scope20/3
  Demux6/2 -> ib_AE1/1
  ia_AE1/1 -> Scope20/1
  vcp_AE2/1 -> Scope10/1
  [Q3] -> Scope18/1, Q_AE1/2
  Q_AE1/1 -> Scope5/2
  [P3] -> P_AE1/2, Scope7/1
  [Vcp1] -> Scope21/2, vcp_AE1/2
  [vcp_pred3] -> Scope21/1, vcp_AE1/1
  [vcn_pred3] -> vcn_AE1/1
  Demux6/3 -> ic_AE1/1
  [Vdc_meas1] -> Scope16/1, vcp_AE2/2
  [Vcn1] -> vcn_AE1/2
  [Vdc_pred3] -> Scope16/2, vcp_AE2/1
  ib_AE1/1 -> Scope20/2
  Step2/1 -> Pstep1/1
  Step4/1 -> 3fault_enable/1
  Step6/1 -> 3fault_enable/2
  Step7/1 -> afault_enable1/1
  Step8/1 -> afault_enable1/2
  3fault_enable/1 -> [enable_3fault]
  afault_enable1/1 -> [enable_afault]
  ka/1 -> [ac_step_a]
  [enable_3fault] -> Gain/1
  Gain/1 -> ka/2
  [enable_afault] -> Gain1/1
  Gain1/1 -> ka/3
  Constant/1 -> ka/1
  kb/1 -> [ac_step_b]
  Constant1/1 -> kb/1
  [enable_3fault] -> Gain2/1
  Gain2/1 -> kb/2
  Step3/1 -> Pstep/2
  Pstep/1 -> [power_step]
  Pstep1/1 -> [dc_step]
  Step5/1 -> Pstep1/2
  Step9/1 -> afault_enable2/1
  Step10/1 -> afault_enable2/2
  afault_enable2/1 -> [enable_edisturb]
  Gain4/1 -> ka/4
  [enable_edisturb] -> Gain4/1
  [enable_edisturb] -> Gain5/1
  Gain5/1 -> kb/3
  [enable_3fault] -> Gain3/1
  Gain3/1 -> kb1/2
  Gain6/1 -> kb1/3
  [enable_edisturb] -> Gain6/1
  kb1/1 -> [ac_step_c]
  Constant2/1 -> kb1/1
  PWM_SPS1/1(Pulse) -> Memory1/1
  Mux16/1 -> MATLAB Function3/1(u)
  [Iabc_Bus_MV3] -> Mux13/2
  [Vabc_Bus_MV3] -> Gain8/1
  Memory1/1 -> [pulses3]
  Product9/1 -> Controlled Voltage Source16/1
  [Iabc_pred3] -> Demux8/1
  [Vref_PQctrl3] -> PWM_SPS1/2(Vref)
  [vcp_pred3] -> Minus1/1
  Bus_1/1 -> [Vabc_Bus_MV3]
  Sine Wave2/1 -> Product2/1
  [pulse_enable] -> Ideal Switch2/1
  Demux9/5 -> Mux15/3  "ic"
  Rec_VQcontrol1/1(V_cell_ref) -> [Vref_PQctrl3]
  Sine Wave9/1 -> Product9/1
  Current Measurement1/1 -> [Idc_Ld5]
  Unary Minus4/1 -> [Iabc_pred3]
  Qref_pu8/1 -> Mux14/2
  Divide6/1 -> [Q3]
  [vcp_pred3] -> Controlled Voltage Source3/1
  [Vdc_pred3] -> Rec_VQcontrol1/3(Vdc)
  [Vabc_Bus_MV3] -> "Power (3ph, Instantaneous)3"/1
  Current Measurement3/1 -> [Idc_Ld6]
  [ac_step_a] -> Product1/2
  [pulse_enable] -> PWM_SPS1/1(enable)
  Demux8/2 -> Controlled Current Source4/1
  [power_step] -> Mux14/1
  [pwmcarrier] -> PWM_SPS1/3(pwmcarrier)
  "Power (3ph, Instantaneous)3"/2 -> Divide6/1
  Demux9/4 -> Mux15/2  "ib"
  [pulses3] -> Mux16/5
  Mux10/1 -> MATLAB Function2/1(u)
  Qref_pu1/1 -> Divide1/2
  Mux14/1 -> Rec_VQcontrol1/2(PQref)
  [ac_step_c] -> Product9/2
  Demux8/1 -> Controlled Current Source5/1
  [Vabc_Bus_MV3] -> Mux13/1
  Minus1/1 -> [Vdc_pred3]
  Qref_pu2/1 -> Divide6/2
  From115/1 -> Gain31/1
  Sine Wave1/1 -> Product1/1
  "Power (3ph, Instantaneous)3"/1 -> Divide1/1
  [Idc_Ld5] -> Gain7/1
  From123/1 -> Mux10/5
  Divide1/1 -> [P3]
  [Q3] -> Scope6/2
  Bus_1/2 -> [Iabc_Bus_MV3]
  [Idc_Ld6] -> Gain9/1
  Demux9/1 -> [vcp_pred3]  "vcp"
  [dc_step] -> Controlled Voltage Source4/1
  Mux13/1 -> Rec_VQcontrol1/1(meas)
  [ac_step_b] -> Product2/2
  [Iabc_Bus_MV3] -> "Power (3ph, Instantaneous)3"/2
  [vcn_pred3] -> Controlled Voltage Source6/1
  From117/1 -> Gain33/1
  Demux9/3 -> Mux15/1  "ia"
  Mux15/1 -> Unary Minus4/1
  MATLAB Function3/1(dz) -> Integrator3/1
  [vcn_pred3] -> Minus1/2
  [P3] -> Scope6/1
  Demux8/3 -> Controlled Current Source6/1
  Product1/1 -> Controlled Voltage Source14/1
  From119/1 -> Gain32/1
  Demux9/2 -> [vcn_pred3]  "vcn"
  Product2/1 -> Controlled Voltage Source15/1
  [Q3] -> Mux12/5
  [Iabc_pred3] -> Mux12/3
  [vcp_pred3] -> Mux12/1
  [Vdc_pred3] -> Mux12/6
  [P3] -> Mux12/4
  [vcn_pred3] -> Mux12/2
  Mux12/1 -> To Workspace2/1
  Gain7/1 -> Mux16/2
  Gain9/1 -> Mux16/3
  Gain8/1 -> Mux16/4
  Integrator3/1 -> Demux10/1
  Demux10/1 -> Gain10/1  "vcp"
  Demux10/2 -> Gain11/1  "vcn"
  Demux10/3 -> Gain12/1  "ia"
  Demux10/4 -> Gain13/1  "ib"
  Demux10/5 -> Gain14/1  "ic"
  Gain10/1 -> Mux17/1
  Gain11/1 -> Mux17/2
  Gain12/1 -> Mux17/3
  Gain13/1 -> Mux17/4
  Gain14/1 -> Mux17/5
  Mux17/1 -> Mux16/1, Demux9/1
  Gain22/1 -> Mux22/3
  [Idc_Ld8] -> Gain22/1
  Demux13/1 -> Controlled Current Source8/1
  [Vabc_Bus_MV4] -> Mux19/1
  [ac_step_c] -> Product12/2
  From129/1 -> Gain39/1
  Qref_pu11/1 -> Divide8/2
  Minus2/1 -> [Vdc_pred4]
  Mux23/1 -> Mux22/1, Demux14/1
  Gain20/1 -> Mux22/2
  "Power (3ph, Instantaneous)4"/2 -> Divide8/1
  Mux18/1 -> MATLAB Function4/1(u)
  Mux20/1 -> Rec_VQcontrol4/2(PQref)
  Bus_4/2 -> [Iabc_Bus_MV4]
  [Q4] -> Scope22/2
  From133/1 -> Gain40/1
  [P4] -> Scope22/1
  Product10/1 -> Controlled Voltage Source17/1
  Demux13/3 -> Controlled Current Source9/1
  [vcn_pred4] -> Minus2/2
  From131/1 -> Gain41/1
  [ac_step_b] -> Product11/2
  Mux19/1 -> Rec_VQcontrol4/1(meas)
  [dc_step] -> Controlled Voltage Source21/1
  [Idc_Ld7] -> Gain20/1
  "Power (3ph, Instantaneous)4"/1 -> Divide7/1
  Sine Wave10/1 -> Product10/1
  From138/1 -> Mux18/5
  PWM_SPS4/1(Pulse) -> Memory4/1
  Demux13/2 -> Controlled Current Source7/1
  [pulse_enable] -> PWM_SPS4/1(enable)
  Current Measurement9/1 -> [Idc_Ld8]
  [pwmcarrier] -> PWM_SPS4/3(pwmcarrier)
  [power_step] -> Mux20/1
  Qref_pu12/1 -> Mux20/2
  [vcp_pred4] -> Controlled Voltage Source20/1
  Product11/1 -> Controlled Voltage Source18/1
  Rec_VQcontrol4/1(V_cell_ref) -> [Vref_PQctrl4]
  Current Measurement5/1 -> [Idc_Ld7]
  [Vref_PQctrl4] -> PWM_SPS4/2(Vref)
  [Vabc_Bus_MV4] -> Gain21/1
  Bus_4/1 -> [Vabc_Bus_MV4]
  Gain21/1 -> Mux22/4
  Product12/1 -> Controlled Voltage Source19/1
  Qref_pu10/1 -> Divide7/2
  Sine Wave11/1 -> Product11/1
  [vcp_pred4] -> Minus2/1
  [vcn_pred4] -> Controlled Voltage Source22/1
  Memory4/1 -> [pulses4]
  [Iabc_pred4] -> Demux13/1
  [pulses4] -> Mux22/5
  [Iabc_Bus_MV4] -> Mux19/2
  [Vdc_pred4] -> Rec_VQcontrol4/3(Vdc)
  [Iabc_Bus_MV4] -> "Power (3ph, Instantaneous)4"/2
  [Vabc_Bus_MV4] -> "Power (3ph, Instantaneous)4"/1
  Sine Wave12/1 -> Product12/1
  [ac_step_a] -> Product10/2
  Mux22/1 -> MATLAB Function5/1(u)
  [pulse_enable] -> Ideal Switch4/1
  Divide8/1 -> [Q4]
  Divide7/1 -> [P4]
  [Q5] -> Scope23/2
  [Idc_Ld9] -> Gain28/1
  [ac_step_b] -> Product14/2
  [dc_step] -> Controlled Voltage Source27/1
  Qref_pu14/1 -> Divide10/2
  Minus3/1 -> [Vdc_pred5]
  MATLAB Function7/1(dz) -> Integrator7/1
  [power_step] -> Mux27/1
  [pwmcarrier] -> PWM_SPS5/3(pwmcarrier)
  [pulse_enable] -> PWM_SPS5/1(enable)
  Current Measurement11/1 -> [Idc_Ld10]
  Demux17/2 -> Controlled Current Source10/1
  From156/1 -> Gain47/1
  [Vabc_Bus_MV5] -> Mux26/1
  Demux17/1 -> Controlled Current Source11/1
  Gain59/1 -> Mux30/5
  Gain58/1 -> Mux30/4
  Gain57/1 -> Mux30/3
  [Idc_Ld10] -> Gain30/1
  Gain30/1 -> Mux29/3
  Demux18/3 -> Mux28/1  "ia"
  Mux28/1 -> Unary Minus8/1
  [vcn_pred5] -> Minus3/2
  Product13/1 -> Controlled Voltage Source23/1
  Mux25/1 -> MATLAB Function6/1(u)
  From158/1 -> Gain49/1
  Qref_pu15/1 -> Mux27/2
  Unary Minus8/1 -> [Iabc_pred5]
  [ac_step_c] -> Product15/2
  [pulse_enable] -> Ideal Switch5/1
  Mux29/1 -> MATLAB Function7/1(u)
  [ac_step_a] -> Product13/2
  [Vabc_Bus_MV5] -> "Power (3ph, Instantaneous)5"/1
  [Iabc_Bus_MV5] -> "Power (3ph, Instantaneous)5"/2
  [Iabc_Bus_MV5] -> Mux26/2
  [vcp_pred5] -> Controlled Voltage Source26/1
  [pulses5] -> Mux29/5
  Memory5/1 -> [pulses5]
  [P5] -> Scope23/1
  [vcp_pred5] -> Minus3/1
  Gain29/1 -> Mux29/4
  Sine Wave15/1 -> Product15/1
  Product15/1 -> Controlled Voltage Source25/1
  Bus_6/1 -> [Vabc_Bus_MV5]
  [Vabc_Bus_MV5] -> Gain29/1
  [Vref_PQctrl5] -> PWM_SPS5/2(Vref)
  [Iabc_pred5] -> Demux17/1
  Sine Wave14/1 -> Product14/1
  Qref_pu13/1 -> Divide9/2
  Current Measurement10/1 -> [Idc_Ld9]
  Divide9/1 -> [P5]
  Divide10/1 -> [Q5]
  Sine Wave13/1 -> Product13/1
  Mux26/1 -> Rec_VQcontrol5/1(meas)
  From165/1 -> Mux25/5
  [Vdc_pred5] -> Rec_VQcontrol5/3(Vdc)
  "Power (3ph, Instantaneous)5"/1 -> Divide9/1
  PWM_SPS5/1(Pulse) -> Memory5/1
  Bus_6/2 -> [Iabc_Bus_MV5]
  Demux18/2 -> [vcn_pred5]  "vcn"
  Gain55/1 -> Mux30/1
  Rec_VQcontrol5/1(V_cell_ref) -> [Vref_PQctrl5]
  Demux18/1 -> [vcp_pred5]  "vcp"
  Mux27/1 -> Rec_VQcontrol5/2(PQref)
  Integrator7/1 -> Demux15/1
  Gain56/1 -> Mux30/2
  Demux18/4 -> Mux28/2  "ib"
  Demux17/3 -> Controlled Current Source12/1
  [vcn_pred5] -> Controlled Voltage Source28/1
  Mux30/1 -> Mux29/1, Demux18/1
  Demux18/5 -> Mux28/3  "ic"
  "Power (3ph, Instantaneous)5"/2 -> Divide10/1
  Product14/1 -> Controlled Voltage Source24/1
  Gain28/1 -> Mux29/2
  [P4] -> Mux32/4
  [vcn_pred4] -> Mux32/2
  [Vdc_pred4] -> Mux32/6
  [Iabc_pred4] -> Mux32/3
  [Q4] -> Mux32/5
  [vcp_pred4] -> Mux32/1
  Mux32/1 -> To Workspace3/1
  [vcp_pred5] -> Mux33/1
  [P5] -> Mux33/4
  Mux33/1 -> To Workspace4/1
  [Q5] -> Mux33/5
  [Iabc_pred5] -> Mux33/3
  [Vdc_pred5] -> Mux33/6
  [vcn_pred5] -> Mux33/2
  [vcp_pred4] -> Scope29/1, vcp_AE3/1
  ib_AE2/1 -> Scope28/2
  Demux20/2 -> ib_AE2/1
  P_AE2/1 -> Scope30/1
  [P1] -> P_AE2/2, Scope31/1
  [Vcp1] -> Scope29/2, vcp_AE3/2
  [Vdc_pred4] -> Scope25/2, vcp_AE4/1
  ic_AE2/1 -> Scope28/3
  Demux20/1 -> Scope32/1, ia_AE2/1
  [Vcn1] -> vcn_AE2/2
  Demux20/3 -> ic_AE2/1
  [Q1] -> Scope26/1, Q_AE2/2
  [Vdc_meas1] -> Scope25/1, vcp_AE4/2
  [Q4] -> Scope26/2, Q_AE2/1
  ia_AE2/1 -> Scope28/1
  Demux19/3 -> ic_AE2/2
  vcn_AE2/1 -> Scope27/2
  Q_AE2/1 -> Scope30/2
  [Iabc_pred4] -> Demux20/1
  vcp_AE4/1 -> Scope24/1
  Demux19/1 -> Scope32/2, ia_AE2/2
  [vcn_pred4] -> vcn_AE2/1
  vcp_AE3/1 -> Scope27/1
  [P4] -> Scope31/2, P_AE2/1
  [Iabc_Bus_MV1] -> Demux19/1
  Demux19/2 -> ib_AE2/2
  Demux21/2 -> ib_AE3/2
  [Iabc_Bus_MV1] -> Demux21/1
  vcp_AE5/1 -> Scope36/1
  Demux21/1 -> Scope41/2, ia_AE3/2
  vcp_AE7/1 -> Scope33/1
  [vcn_pred5] -> vcn_AE3/1
  Demux21/3 -> ic_AE3/2
  [Q5] -> Scope35/2, Q_AE3/1
  Q_AE3/1 -> Scope39/2
  vcn_AE3/1 -> Scope36/2
  [Q1] -> Scope35/1, Q_AE3/2
  [Vdc_meas1] -> Scope34/1, vcp_AE7/2
  [Vcn1] -> vcn_AE3/2
  [Iabc_pred5] -> Demux22/1
  Demux22/3 -> ic_AE3/1
  [Vcp1] -> Scope38/2, vcp_AE5/2
  [Vdc_pred5] -> Scope34/2, vcp_AE7/1
  ic_AE3/1 -> Scope37/3
  [P5] -> Scope40/2, P_AE3/1
  Demux22/1 -> Scope41/1, ia_AE3/1
  ia_AE3/1 -> Scope37/1
  [vcp_pred5] -> Scope38/1, vcp_AE5/1
  P_AE3/1 -> Scope39/1
  Demux22/2 -> ib_AE3/1
  ib_AE3/1 -> Scope37/2
  [P1] -> P_AE3/2, Scope40/1
  Gain31/1 -> Mux10/2
  Gain32/1 -> Mux10/4
  Gain33/1 -> Mux10/3
  Gain41/1 -> Mux18/3
  Gain39/1 -> Mux18/2
  Gain40/1 -> Mux18/4
  Gain47/1 -> Mux25/2
  Gain49/1 -> Mux25/3
  From160/1 -> Gain48/1
  Gain48/1 -> Mux25/4
  Gain36/1 -> Mux34/3
  Gain37/1 -> Mux34/4
  Gain38/1 -> Mux34/5
  Mux34/1 -> Mux10/1, Demux23/1
  Demux23/4 -> Mux9/2  "ib"
  Gain35/1 -> Mux34/2
  Gain34/1 -> Mux34/1
  Demux23/2 -> Goto13/1  "vcn"
  Demux7/5 -> Gain38/1  "ic"
  Demux23/1 -> Goto12/1  "vcp"
  Mux9/1 -> Unary Minus3/1
  Demux23/3 -> Mux9/1  "ia"
  Integrator2/1 -> Demux7/1
  Unary Minus3/1 -> Goto2/1
  Demux23/5 -> Mux9/3  "ic"
  MATLAB Function2/1(dz) -> Integrator2/1
  Demux7/1 -> Gain34/1  "vcp"
  Demux7/4 -> Gain37/1  "ib"
  Demux7/3 -> Gain36/1  "ia"
  Demux7/2 -> Gain35/1  "vcn"
  MATLAB Function4/1(z_next) -> Unit Delay1/1
  Demux12/1 -> Gain42/1  "vcp"
  Demux12/4 -> Gain45/1  "ib"
  Demux12/2 -> Gain43/1  "vcn"
  Demux12/3 -> Gain44/1  "ia"
  Gain42/1 -> Mux35/1
  Gain46/1 -> Mux35/5
  Gain44/1 -> Mux35/3
  Gain45/1 -> Mux35/4
  Demux24/3 -> Mux24/1  "ia"
  Mux24/1 -> Unary Minus5/1
  Demux24/2 -> Goto61/1  "vcn"
  Unary Minus5/1 -> Goto55/1
  Demux24/1 -> Goto56/1  "vcp"
  Demux24/4 -> Mux24/2  "ib"
  Demux12/5 -> Gain46/1  "ic"
  Unit Delay1/1 -> Demux12/1
  Gain43/1 -> Mux35/2
  Demux24/5 -> Mux24/3  "ic"
  Mux35/1 -> Mux18/1, Demux24/1
  MATLAB Function5/1(z_next) -> Unit Delay/1
  Unit Delay/1 -> Demux11/1
  Demux14/1 -> [vcp_pred4]  "vcp"
  Demux14/2 -> [vcn_pred4]  "vcn"
  Demux14/3 -> Mux21/1  "ia"
  Demux14/4 -> Mux21/2  "ib"
  Demux14/5 -> Mux21/3  "ic"
  Mux21/1 -> Unary Minus6/1
  Unary Minus6/1 -> [Iabc_pred4]
  Demux11/1 -> Gain15/1  "vcp"
  Demux11/2 -> Gain16/1  "vcn"
  Demux11/3 -> Gain17/1  "ia"
  Demux11/4 -> Gain18/1  "ib"
  Demux11/5 -> Gain19/1  "ic"
  Gain15/1 -> Mux23/1
  Gain16/1 -> Mux23/2
  Gain17/1 -> Mux23/3
  Gain18/1 -> Mux23/4
  Gain19/1 -> Mux23/5
  Demux15/1 -> Gain55/1  "vcp"
  Demux15/2 -> Gain56/1  "vcn"
  Demux15/3 -> Gain57/1  "ia"
  Demux15/4 -> Gain58/1  "ib"
  Demux15/5 -> Gain59/1  "ic"
  Demux16/3 -> Gain25/1  "ia"
  Mux31/1 -> Unary Minus7/1
  Demux25/3 -> Mux31/1  "ia"
  Integrator4/1 -> Demux16/1
  Demux25/1 -> Goto72/1  "vcp"
  Demux16/2 -> Gain24/1  "vcn"
  Demux16/4 -> Gain26/1  "ib"
  Demux25/2 -> Goto76/1  "vcn"
  Demux16/5 -> Gain27/1  "ic"
  Demux16/1 -> Gain23/1  "vcp"
  Mux36/1 -> Mux25/1, Demux25/1
  Unary Minus7/1 -> Goto71/1
  Demux25/5 -> Mux31/3  "ic"
  Gain26/1 -> Mux36/4
  Gain24/1 -> Mux36/2
  Gain25/1 -> Mux36/3
  Demux25/4 -> Mux31/2  "ib"
  Gain27/1 -> Mux36/5
  Gain23/1 -> Mux36/1
  MATLAB Function6/1(dz) -> Integrator4/1
  connections:
  Bus_2/RConn2 -- Controlled Voltage Source8/RConn1
  Bus_2/RConn3 -- Controlled Voltage Source9/RConn1
  Bus_2/RConn1 -- Controlled Voltage Source7/RConn1
  Current Measurement2/LConn1 -- Ideal Switch1/LConn1
  Ideal Switch1/RConn1 -- Series RLC Branch2/RConn1
  Current Measurement2/RConn1 -- Controlled Voltage Source1/RConn1
  Current Measurement4/RConn1 -- Controlled Voltage Source2/LConn1
  Controlled Voltage Source5/RConn1 -- Ground4/LConn1 -- Controlled Voltage Source1/LConn1
  Controlled Voltage Source5/LConn1 -- Current Measurement4/LConn1
  Controlled Voltage Source2/RConn1 -- Series RLC Branch2/LConn1
  Controlled Current Source2/LConn1 -- Ground3/LConn1 -- Controlled Current Source3/LConn1 -- Controlled Current Source1/LConn1
  Controlled Current Source2/RConn1 -- Bus_2/LConn1
  Controlled Current Source1/RConn1 -- Bus_2/LConn2
  Bus_2/LConn3 -- Controlled Current Source3/RConn1
  Ground2/LConn1 -- Controlled Voltage Source9/LConn1 -- Controlled Voltage Source7/LConn1 -- Controlled Voltage Source8/LConn1
  Current Measurement8/LConn1 -- IGBT Inverter2/RConn2 -- Voltage Measurement3/LConn2 -- Series RLC Branch3/RConn1 -- Voltage Measurement2/LConn2
  Series RLC Branch5/RConn1 -- Voltage Measurement1/LConn2 -- Ground6/LConn1 -- Series RLC Branch3/LConn1 -- Voltage Measurement2/LConn1
  Series RLC Branch5/LConn1 -- Voltage Measurement3/LConn1 -- Current Measurement6/RConn1 -- Current Measurement7/RConn1 -- Voltage Measurement1/LConn1
  Controlled Voltage Source12/LConn1 -- Ground5/LConn1 -- Controlled Voltage Source13/LConn1 -- Controlled Voltage Source11/LConn1
  Bus_3/LConn2 -- Three-Phase RL1/LConn2
  Current Measurement7/LConn1 -- Ideal Switch3/LConn1
  Bus_3/LConn3 -- Three-Phase RL1/LConn3
  Three-Phase RL1/RConn1 -- Bus_5/RConn1
  Controlled Voltage Source10/RConn1 -- Series RLC Branch4/LConn1
  Ideal Switch3/RConn1 -- Series RLC Branch4/RConn1
  Bus_5/LConn3 -- IGBT Inverter2/LConn3
  Three-Phase RL1/RConn2 -- Bus_5/RConn2
  IGBT Inverter2/RConn1 -- Current Measurement6/LConn1
  Bus_5/LConn1 -- IGBT Inverter2/LConn1
  Controlled Voltage Source12/RConn1 -- Bus_3/RConn2
  Current Measurement8/RConn1 -- Controlled Voltage Source10/LConn1
  Bus_5/LConn2 -- IGBT Inverter2/LConn2
  Three-Phase RL1/RConn3 -- Bus_5/RConn3
  Bus_3/LConn1 -- Three-Phase RL1/LConn1
  Controlled Voltage Source11/RConn1 -- Bus_3/RConn1
  Controlled Voltage Source13/RConn1 -- Bus_3/RConn3
  Controlled Voltage Source15/LConn1 -- Controlled Voltage Source16/LConn1 -- Controlled Voltage Source14/LConn1 -- Ground1/LConn1
  Controlled Voltage Source3/LConn1 -- Controlled Voltage Source6/RConn1 -- Ground8/LConn1
  Controlled Current Source4/LConn1 -- Controlled Current Source5/LConn1 -- Ground7/LConn1 -- Controlled Current Source6/LConn1
  Current Measurement3/RConn1 -- Controlled Voltage Source4/LConn1
  Bus_1/RConn1 -- Controlled Voltage Source14/RConn1
  Controlled Current Source5/RConn1 -- Bus_1/LConn1
  Bus_1/RConn2 -- Controlled Voltage Source15/RConn1
  Controlled Voltage Source6/LConn1 -- Current Measurement3/LConn1
  Bus_1/LConn3 -- Controlled Current Source6/RConn1
  Current Measurement1/RConn1 -- Controlled Voltage Source3/RConn1
  Controlled Current Source4/RConn1 -- Bus_1/LConn2
  Bus_1/RConn3 -- Controlled Voltage Source16/RConn1
  Controlled Voltage Source4/RConn1 -- Series RLC Branch1/LConn1
  Current Measurement1/LConn1 -- Ideal Switch2/LConn1
  Ideal Switch2/RConn1 -- Series RLC Branch1/RConn1
  Controlled Voltage Source18/LConn1 -- Ground9/LConn1 -- Controlled Voltage Source19/LConn1 -- Controlled Voltage Source17/LConn1
  Controlled Voltage Source20/LConn1 -- Controlled Voltage Source22/RConn1 -- Ground11/LConn1
  Controlled Current Source7/LConn1 -- Controlled Current Source8/LConn1 -- Ground10/LConn1 -- Controlled Current Source9/LConn1
  Current Measurement5/LConn1 -- Ideal Switch4/LConn1
  Bus_4/RConn3 -- Controlled Voltage Source19/RConn1
  Controlled Voltage Source21/RConn1 -- Series RLC Branch6/LConn1
  Controlled Current Source7/RConn1 -- Bus_4/LConn2
  Ideal Switch4/RConn1 -- Series RLC Branch6/RConn1
  Controlled Current Source8/RConn1 -- Bus_4/LConn1
  Controlled Voltage Source22/LConn1 -- Current Measurement9/LConn1
  Current Measurement5/RConn1 -- Controlled Voltage Source20/RConn1
  Bus_4/LConn3 -- Controlled Current Source9/RConn1
  Bus_4/RConn2 -- Controlled Voltage Source18/RConn1
  Bus_4/RConn1 -- Controlled Voltage Source17/RConn1
  Current Measurement9/RConn1 -- Controlled Voltage Source21/LConn1
  Controlled Voltage Source26/LConn1 -- Controlled Voltage Source28/RConn1 -- Ground13/LConn1
  Controlled Voltage Source24/LConn1 -- Ground14/LConn1 -- Controlled Voltage Source25/LConn1 -- Controlled Voltage Source23/LConn1
  Controlled Current Source10/LConn1 -- Controlled Current Source11/LConn1 -- Ground12/LConn1 -- Controlled Current Source12/LConn1
  Current Measurement10/LConn1 -- Ideal Switch5/LConn1
  Bus_6/RConn1 -- Controlled Voltage Source23/RConn1
  Controlled Voltage Source28/LConn1 -- Current Measurement11/LConn1
  Bus_6/LConn3 -- Controlled Current Source12/RConn1
  Current Measurement10/RConn1 -- Controlled Voltage Source26/RConn1
  Bus_6/RConn2 -- Controlled Voltage Source24/RConn1
  Controlled Current Source10/RConn1 -- Bus_6/LConn2
  Bus_6/RConn3 -- Controlled Voltage Source25/RConn1
  Controlled Current Source11/RConn1 -- Bus_6/LConn1
  Current Measurement11/RConn1 -- Controlled Voltage Source27/LConn1
  Controlled Voltage Source27/RConn1 -- Series RLC Branch7/LConn1
  Ideal Switch5/RConn1 -- Series RLC Branch7/RConn1

== system AI_Compare_2level/Help ==

== system AI_Compare_2level/Model Initialization ==
